simulink model "psbtransient8"  (Simulink 5.0)
settings: Solver=ode23tb  SolverMode=SingleTasking  StartTime=0.0  StopTime=0.2  RelTol=1e-3
libraries: powerlib2 x17
settings Model: Creator=patrice  LastModifiedBy=User  ExtModeTrigMode=oneshot  ExtModeArmWhenConnect=off  LimitDataPoints=off  BlockReductionOpt=off  BooleanDataType=off  RTWTemplateMakefile=grt_unix.tmf

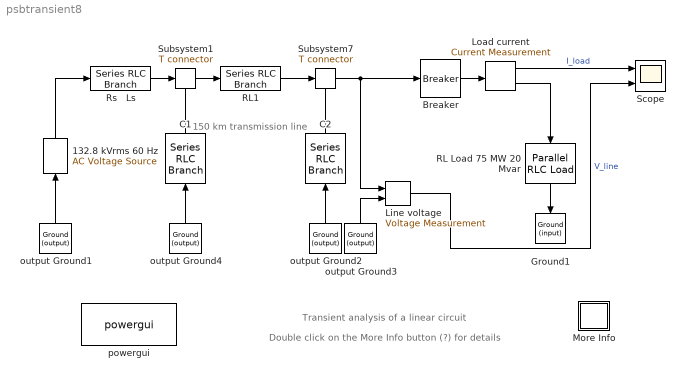
== system psbtransient8 ==
  note: Double click on the More Info button (?) for details
  note: Transient analysis of a linear circuit
  note: 150 km
      | transmission line
  132.8 kVrms 60 Hz : powerlib2/Electrical Sources/AC Voltage Source  Tag=PoWeRsYsTeMbLoCk  Orientation=up  A=230e3/sqrt(3)*sqrt(2)  P=90  F=60  stime=0  mesure=None  PSBOutputType=1
  Breaker : powerlib2/Elements/Breaker  Tag=PoWeRsYsTeMbLoCk  a=0.01  c=1  rs=inf  cs=0  times="[ 2/60  7/60 ]"  Ts=0  comext=off  mesure=None  PSBOutputType=1
  C1 : powerlib2/Elements/Series RLC Branch  Tag=PoWeRsYsTeMbLoCk  Orientation=up  a=0  b=0  c=0.967e-06  mesure=None  PSBOutputType=1
  C2 : powerlib2/Elements/Series RLC Branch  Tag=PoWeRsYsTeMbLoCk  Orientation=up  a=0  b=0  c=0.967e-06  mesure=None  PSBOutputType=1
  Ground1 : powerlib2/Connectors/Ground (input)  Tag=PoWeRsYsTeMbLoCk  Orientation=down
  Line voltage : powerlib2/Measurements/Voltage Measurement  Tag=PoWeRsYsTeMmEaSuReMeNt  PhasorSimulation=off  OutputType=Magnitude  PSBOutputType=0  PSBequivalent=0
  Load current : powerlib2/Measurements/Current Measurement  Tag=PoWeRsYsTeMmEaSuReMeNt  PhasorSimulation=off  OutputType=Magnitude  PSBOutputType=01  PSBequivalent=1
  More Info : Subsystem
      mask Display: disp('?')
  RL Load 75 MW 20 Mvar : powerlib2/Elements/Parallel RLC Load  Tag=PoWeRsYsTeMbLoCk  Orientation=down  a=132.8e3  b=60  c=75e6  d=20e6  e=0  mesure=None  PSBOutputType=1
  RL1 : powerlib2/Elements/Series RLC Branch  Tag=PoWeRsYsTeMbLoCk  a=5.2  b=138e-3  c=inf  mesure=None  PSBOutputType=1
  Rs   Ls : powerlib2/Elements/Series RLC Branch  Tag=PoWeRsYsTeMbLoCk  a=2.645  b=70.2e-03  c=inf  mesure=None  PSBOutputType=1
  Scope : Scope  NumInputPorts=2
      settings: TimeRange=0.2  YMin=-1000~-400000  YMax=1000~400000  DataFormat=Array
  Subsystem1 : powerlib2/Connectors/T connector  Tag=PoWeRsYsTeMbLoCk  PSBOutputType=1
  Subsystem7 : powerlib2/Connectors/T connector  Tag=PoWeRsYsTeMbLoCk  PSBOutputType=1
  output Ground{1..4} (4 alike) : powerlib2/Connectors/Ground (output)  Tag=PoWeRsYsTeMbLoCk  Orientation=up  PSBOutputType=1
  powergui : powerlib2/powergui  Frange=logspace(0,3,50)  Ylog=off  Xlog=off  save=off  variable=ZData  ZoomFFT=on  StartTime=0.0  cycles=1  DisplayStyle=off  fundamental=60  FreqAxis=off  MaxFrequency=1000  frequencyindice=1  frequencyindicesteady=1  RmsSteady=1  display=off  Ts=0  methode=off  frequency=60  echomessages=off
  wires:
  RL Load 75 MW 20 Mvar/1 -> Ground1/1
  output Ground3/1 -> Line voltage/2
  Subsystem7/1 -> Line voltage/1, Breaker/1
  output Ground2/1 -> C2/1
  C2/1 -> Subsystem7/Enable
  RL1/1 -> Subsystem7/1
  132.8 kVrms 60 Hz/1 -> Rs   Ls/1
  output Ground1/1 -> 132.8 kVrms 60 Hz/1
  Line voltage/1 -> Scope/2  "V_line"
  Load current/1 -> Scope/1  "I_load"
  Breaker/1 -> Load current/1
  Load current/2 -> RL Load 75 MW 20 Mvar/1
  Rs   Ls/1 -> Subsystem1/1
  Subsystem1/1 -> RL1/1
  C1/1 -> Subsystem1/Enable
  output Ground4/1 -> C1/1

== system psbtransient8/More Info ==
  note: This demonstration illustrates steady-state and transient simulation of a linear circuit and use of the Powergui block
  note: Circuit Description
  note: This circuit is a simplified model of a 230 kV  three-phase power system. Only one phase of the transmission system is represented.
      | The equivalent source is modeled by a voltage source (230 kV rms/sqrt(3) or 187.8 kV peak, 60 Hz) in series with its  internal impedance (Rs Ls)
      | corresponding to  a 3-phase 2000 MVA short circuit level and X/R = 10. (X = 230e3^2/2000e6 = 26.45 ohms or L = 0.0702 H, R = X/10 = 2.645 ohms).
      | The source feeds a RL load through a 150 km transmission line. The line distributed parameters  (R = 0.035ohm/km, L = 0.92 mH/km, C = 12.9 nF/km)
      |  are modeled by a single pi section (RL1 branch 5.2 ohm; 138 mH  and  two shunt capacitances  C1 and C2 of  0.967 uF).
      | The load (75 MW -20 Mvar per phase) is modeled by a parallel RLC load block.
      |
      | A circuit breaker is used to switch the load at  the receiving end of the transmission line. The breaker which is initially  closed is opened at t = 2 cycles,
      | then it is reclosed at t = 7 cycles. Current and Voltage Measurement blocks provide signals for visualization purpose.
  note: H. Le-Huy (Université Laval, Québec) and G. Sybille (Hydro-Québec)
  note: Start the simulation and observe  line voltage and  load current  transients during  load switching and note that the simulation starts in steady-state.
      | Use the zoom buttons of the oscilloscope to observe the transient voltage at breaker reclosing.
  note: 1. Simulation using a continuous solver (ode23tb)
  note: Open the Powergui block and select "Steady State Voltage and Currents" to measure the steady-state  voltage and current  phasors.
      |
      | Using the Powergui select now  "Initial  States Setting"  to obtain the initial state values (voltage across capacitors and current in inductances).
      | Now, reset all the initial states to zero by clicking the  "to zero" button and then "Apply" to confirm changes. Restart the simulation and observe  transients
      | at simulation starting. Using the same Powergui window, you can also set selected states to specific values.
  note: 2. Using the powergui to obtain steady-state phasors and set initial states
  note: 3. Discretizing your circuit and simulating at fixed steps
  note: The Powergui block can also be used to  discretize your circuit and simulate it at fixed steps.
      |
      | Open the Powergui . Select  "Discretize electrical model" and specify a sample time of 50e-6 s. The state-space model will now be discretized
      | using trapezoidal fixed step integration. The precision of results is now imposed by the sample time. Restart the simulation and compare simultion results
      | with the continuous integration method.  Vary the sample time of the discrete system and note the impact on precision of fast transients.
  note: 4. Using the phasor simulation method
  note: You will now use a third simulation technique.  The "phasor simulation" method consists to replace the circuit state-space model by a set of algebraic
      | equations evaluated at a fixed frequency and to replace sinusoidal voltage and current sources by phasors (complex numbers). This method allows a fast
      | computation of voltage and current phasors at a selected frequency, disregarding fast transients. It is particularly efficient to study electromechanical
      | transients of generators and motors involving low frequency oscillation modes.
      |
      | Open  the Powergui  block and select "Phasor simulation". Restart the simulation. Observe that the magnitude of 60 Hz  voltage and current is now displayed
      | on the scope. If you double click on the  voltage or current measurement block you can choose to output phasor signals in four different formats:
      | Complex, Real/Imag, Magnitude/Angle (in degres),  or just Magnitude (default value). Notice that you cannot send a complex signal to an oscilloscope.
  note: Demonstration
